simulink model "behinehsazy_nonLinear"  (R2018b)
settings: Solver=VariableStepAuto  StartTime=0.0  StopTime=1  RelTol=1e-3
values from neighbouring files (symbols this model uses):
  A = double(A)    [Linearization.m]    (also in findK_emtiazi.m = [1 2 0; 0 -1 3; 0 1 -1])
  B = double(B)    [Linearization.m]
  C = [1 0 0 0 ; 0 1 0 0 ]    [Linearization.m]    (also in findK_emtiazi.m = [0 1 0])
  k1 = double(k1)    [Linearization.m]
settings Model: Creator=sepehr  LastModifiedBy=sepehr

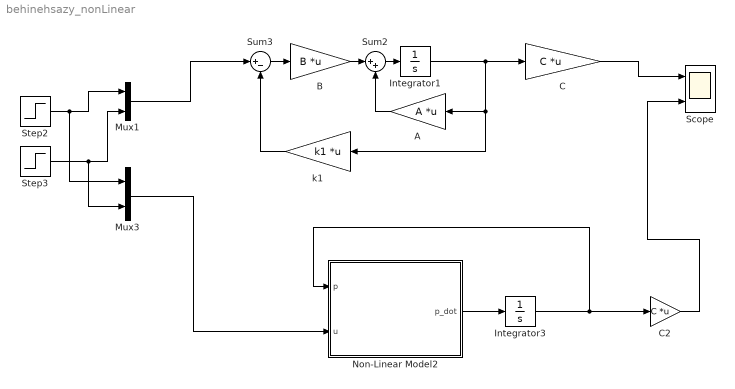
== system behinehsazy_nonLinear ==
  "A " : Gain  Gain=A  Multiplication=Matrix(K*u) (u vector)
  B : Gain  Gain=B  Multiplication=Matrix(K*u) (u vector)
  C : Gain  Gain=C  Multiplication=Matrix(K*u) (u vector)
  C2 : Gain  Gain=C  Multiplication=Matrix(K*u) (u vector)
  Integrator1 : Integrator  InitialCondition=[0.5;0.5;0.005;0.008]  IgnoreLimit=on
  Integrator3 : Integrator  InitialCondition=zeros(4,1)
  Mux1 : Mux  Inputs=2
  Mux3 : Mux  Inputs=2
  Non-Linear Model2 : MATLAB Function  TreatAsAtomicUnit=on
  Scope : Scope  NumInputPorts=2
  Step2 : Step  After=100  SampleTime=0.1
  Step3 : Step  After=100  SampleTime=0.1
  Sum2 : Sum  Inputs=|++
  Sum3 : Sum  Inputs=|+-
  "k1 " : Gain  Gain=k1  Multiplication=Matrix(K*u) (u vector)
  wires:
  Sum3/1 -> B/1
  Mux1/1 -> Sum3/1
  Step2/1 -> Mux3/1, Mux1/1
  "A "/1 -> Sum2/2
  Sum2/1 -> Integrator1/1
  Step3/1 -> Mux1/2, Mux3/2
  "k1 "/1 -> Sum3/2
  B/1 -> Sum2/1
  Integrator1/1 -> C/1, "A "/1, "k1 "/1
  C/1 -> Scope/1
  Mux3/1 -> Non-Linear Model2/2(u)
  Non-Linear Model2/1(p_dot) -> Integrator3/1
  Integrator3/1 -> Non-Linear Model2/1(p), C2/1
  C2/1 -> Scope/2

== matlab function behinehsazy_nonLinear/Non-Linear Model2 ==
  data: p input; u input; p_dot output
function p_dot = fcn(p,u)

a1 = 6.11e-3;
a2 = -2.89e-3;
a3 = -4.24e-3;
a4 = 3.01e-3;
a5 = 2.05e-3;
a6 = 1.92e-3;
a7 = 1.60e-3;
a8 = -8.32e-3;
bw = 30;
cw = 1500;
d1 = 0;
d2 = 0;

p1 = p(1);
p2 = p(2);
p3 = p(3);
p4 = p(4);

M = [a1 + a2*cos(2*p2) + a3*sin(2*p2) + a4*cos(p2) + a5*sin(p2) 0; 0 a6];
M_inv = inv(M);
V = [-2*a1*p3*p4*sin(2*p2) + 2*a3*p3*p4*cos(2*p2) + a4*p3*p4*cos(p2) - a5*p3*p4*sin(p2) ; 
    2*a2*(p3)^2*cos(p2)*sin(p2) - a3*(p3)^2*cos(p2) - 0.5*a4*(p3)^2*cos(p2) + 0.5*a5*(p3)^2*sin(p2) + a7*sin(p2) + a8*cos(p2)];
f = bw*[p3;p4] + cw*[p1;p2];
%u = [u1 ; u2];
d = [d1 ; d2];
C = [1 0 0 0 ; 0 1 0 0 ];


x1_dot = [p3 ; p4];
x2_dot = -M_inv*V - M_inv*f + M_inv*u + M_inv*d;

p_dot = [x1_dot ; x2_dot];
